simulink subsystem "VehicleDynamics"  (R2023b)
settings: Solver=VariableStepAuto  StartTime=0.0  StopTime=10.0  RelTol=1e-3
undefined symbols (not defined in the file or in its folder): accMAX, brakeMAX, jerkMAX, lr, m, position0, turnAngleMAX, turnAngleRateMAX, velocity0
libraries: autolibshared x1
settings Model: Creator=Victor  LastModifiedBy=Victor

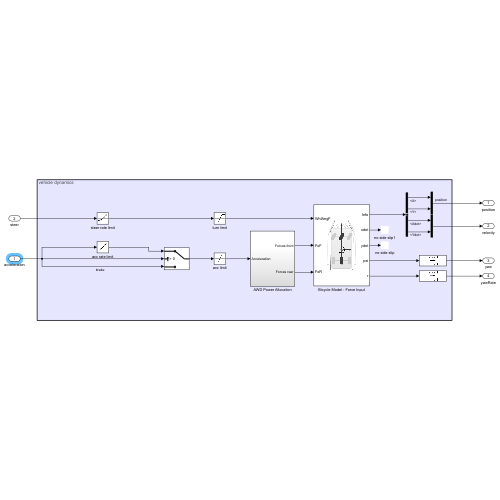
[thumbnail: Simulink's stored preview of the top-level diagram]
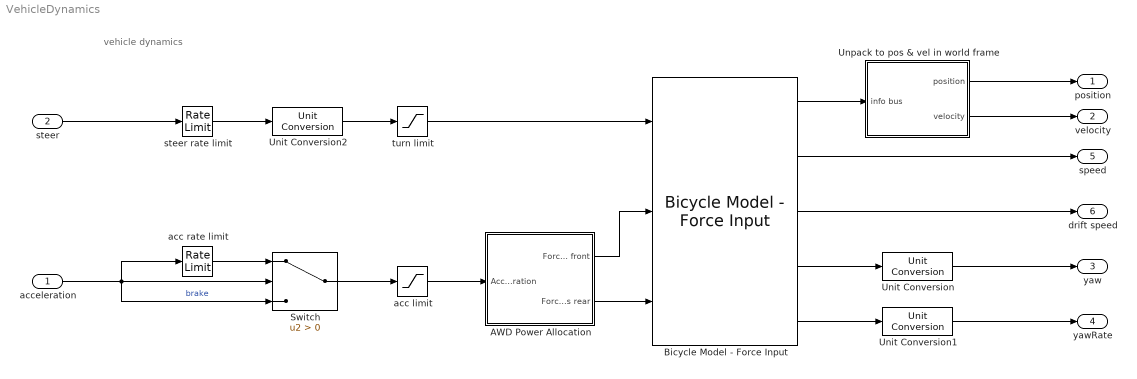
== system VehicleDynamics ==
  note: vehicle dynamics
  acceleration : Inport  Unit=m/s^2  PortDimensions=1
  steer : Inport  Port=2  Unit=deg  PortDimensions=1
  AWD Power Allocation : Subsystem
  Bicycle Model - Force Input : autolibshared/Bicycle Model - Force Input  trackMode=Single (bicycle)  inputMode=External longitudinal forces  frontSteerMode=on  rearSteerMode=off  windMode=off  muMode=off  extFMode=off  extMMode=off  aMode=3  NF=2  NR=2  m=m  a=lf  b=lr  h=0.35  X_o=position0(1)  xdot_o=velocity0(1)  CalphaMode=off  sigmaMode=on  w=[1.4,1.4]  Cy_f=Cf  Cy_r=Cr  sigma_f=.1  sigma_r=.1  alpha_f_brk=[-.1 .1]  Cy_f_data=[-9e3 9e3]  alpha_r_brk=[-.1 .1]  Cy_r_data=[-9e3 9e3]  Y_o=position0(2)  ydot_o=velocity0(2)  Izz=Iz  psi_o=yaw0  r_o=yawRate0  Af=0  Cd=.3  Cl=.1  Cpm=.1  beta_w=[0:0.01:0.3]  Cs=[0:0.03:0.9]  Cym=[0:0.01:0.3]  Pabs=101325  Tair=273  g=9.81  mu=1  xdot_tol=.01  Fznom=5000  Fxtire_sat=1e6  Fytire_sat=1e6  longOff=0  latOff=0  vertOff=0
      settings: LibrarySourceBlock=drivingscenarioandsensors/Bicycle Model - Force Input
  Switch : Switch  Criteria=u2 > Threshold  SaturateOnIntegerOverflow=off  InputSameDT=off
  Unit Conversion : UnitConversion  OutputType=Inherit: Inherit via back propagation
  Unit Conversion1 : UnitConversion  OutputType=Inherit: Inherit via back propagation
  Unit Conversion2 : UnitConversion  OutputType=Inherit: Inherit via back propagation
  Unpack to pos & vel in world frame : Subsystem
  acc limit : Saturate  UpperLimit=accMAX  LowerLimit=-brakeMAX
  acc rate limit : RateLimiter  RisingSlewLimit=jerkMAX  FallingSlewLimit=-jerkMAX  SampleTimeMode=inherited
  steer rate limit : RateLimiter  RisingSlewLimit=turnAngleRateMAX  FallingSlewLimit=-turnAngleRateMAX  SampleTimeMode=inherited
  turn limit : Saturate  UpperLimit=turnAngleMAX  LowerLimit=-turnAngleMAX
  position : Outport  Unit=m  PortDimensions=2
  velocity : Outport  Port=2  Unit=m/s  PortDimensions=2
  yaw : Outport  Port=3  Unit=deg  PortDimensions=1
  yawRate : Outport  Port=4  Unit=deg/s  PortDimensions=1
  speed : Outport  Port=5  Unit=m/s  PortDimensions=1
  drift speed : Outport  Port=6  Unit=m/s  PortDimensions=1
  wires:
  Unit Conversion/1 -> yaw/1
  Unit Conversion1/1 -> yawRate/1
  acc rate limit/1 -> Switch/1
  steer/1 -> steer rate limit/1
  turn limit/1 -> Bicycle Model - Force Input/1
  Switch/1 -> acc limit/1
  acc limit/1 -> AWD Power Allocation/1(Acceleration)
  AWD Power Allocation/2(Forces rear) -> Bicycle Model - Force Input/3
  Bicycle Model - Force Input/3 -> drift speed/1
  Bicycle Model - Force Input/5 -> Unit Conversion1/1
  Bicycle Model - Force Input/4 -> Unit Conversion/1
  acceleration/1 -> acc rate limit/1, Switch/3, Switch/2  "brake"
  Bicycle Model - Force Input/2 -> speed/1
  AWD Power Allocation/1(Forces front) -> Bicycle Model - Force Input/2
  Bicycle Model - Force Input/1 -> Unpack to pos & vel in world frame/1(info bus)
  Unpack to pos & vel in world frame/1(position) -> position/1
  Unpack to pos & vel in world frame/2(velocity) -> velocity/1
  steer rate limit/1 -> Unit Conversion2/1
  Unit Conversion2/1 -> turn limit/1

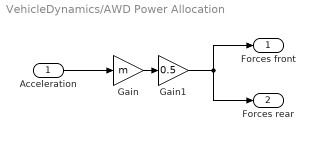
== system VehicleDynamics/AWD Power Allocation ==
  Acceleration : Inport
  Gain : Gain  Gain=m
  Gain1 : Gain  Gain=0.5
  Forces front : Outport  VectorParamsAs1DForOutWhenUnconnected=off
  Forces rear : Outport  Port=2  VectorParamsAs1DForOutWhenUnconnected=off
  wires:
  Gain/1 -> Gain1/1
  Gain1/1 -> Forces front/1, Forces rear/1
  Acceleration/1 -> Gain/1

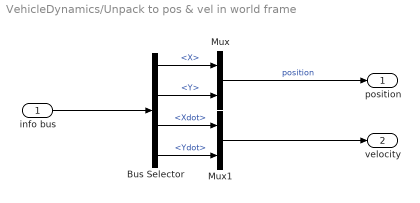
== system VehicleDynamics/Unpack to pos & vel in world frame ==
  info bus : Inport
  Bus Selector : BusSelector  OutputSignals=InertFrm.FrntAxl.Disp.X,InertFrm.FrntAxl.Disp.Y,InertFrm.FrntAxl.Vel.Xdot,InertFrm.FrntAxl.Vel.Ydot
  Mux : Mux  Inputs=2
  Mux1 : Mux  Inputs=2
  position : Outport
  velocity : Outport  Port=2
  wires:
  Mux/1 -> position/1  "position"
  Mux1/1 -> velocity/1
  Bus Selector/2 -> Mux/2  "<Y>"
  Bus Selector/4 -> Mux1/2  "<Ydot>"
  Bus Selector/3 -> Mux1/1  "<Xdot>"
  Bus Selector/1 -> Mux/1  "<X>"
  info bus/1 -> Bus Selector/1
